simulink model "dual_RigidBodyDynamics"  (R2016a)
settings: Solver=VariableStepAuto  StartTime=0  StopTime=10  FixedStep=1  RelTol=1e-3
settings Model: Creator=viav_gi  LastModifiedBy=shriyahazra

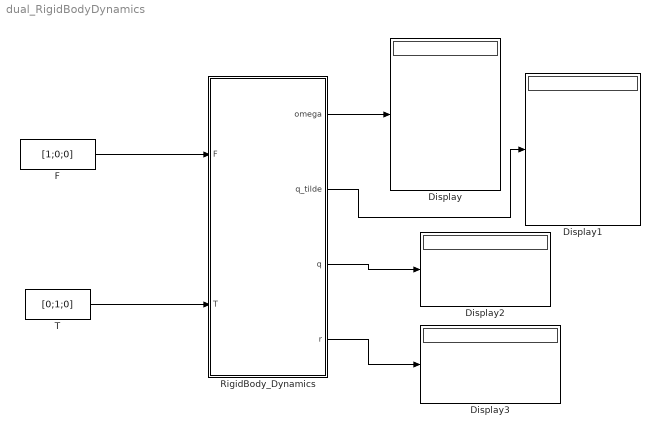
== system dual_RigidBodyDynamics ==
  Display{,1..3} (4 alike) : Display
  F : Constant  Value=[1;0;0]  VectorParams1D=off
  RigidBody_Dynamics : Subsystem  mask{r0=[0;0;0], v0=[0;0;0], m0=1, q0=[0;0;0;1], w0=[0;0;0], J0=eye(3)}
      mask prompts: r0 "Initial position (m) in inertial reference frame, [3,1]"; v0 "Initial velocity (m/s) in inertial reference frame, [3,1]"; m0 "Initial mass (kg), [1,1]"; q0 "Initial quaternion defining the orientation in body reference frame [4,1]"; w0 "Initial angular velocity (rad/s) in body reference frame, [3,1]"; J0 "Initial Inertia matrix (kg*m2),  [3,3]"
  T : Constant  Value=[0;1;0]  VectorParams1D=off
  wires:
  T/1 -> RigidBody_Dynamics/2(T)
  RigidBody_Dynamics/1(omega) -> Display/1
  RigidBody_Dynamics/2("q_tilde ") -> Display1/1
  RigidBody_Dynamics/3(q) -> Display2/1
  RigidBody_Dynamics/4(r) -> Display3/1
  F/1 -> RigidBody_Dynamics/1(F)

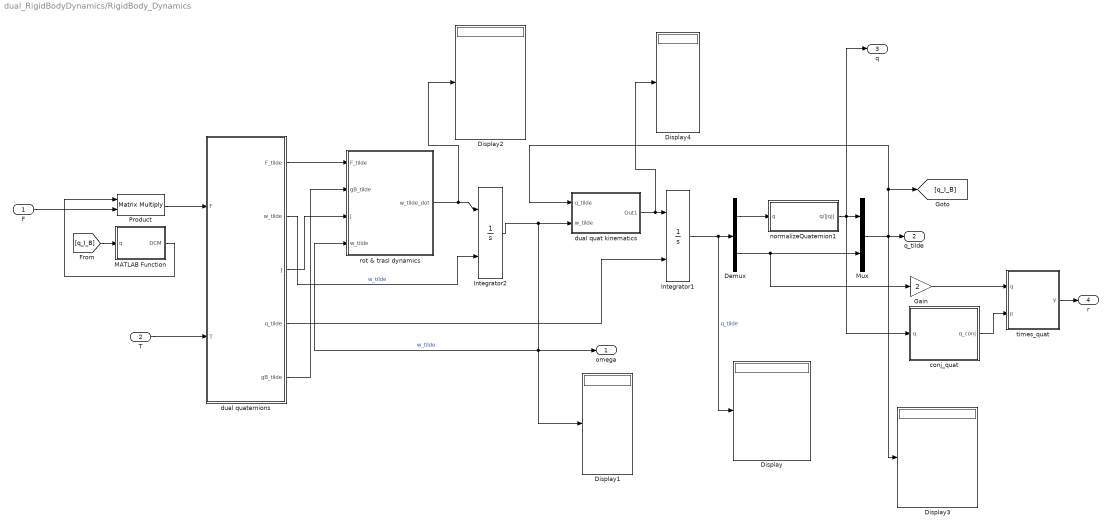
== system dual_RigidBodyDynamics/RigidBody_Dynamics ==
  F : Inport
  T : Inport  Port=2
  Demux : Demux  Outputs=2
  Display{,1..4} (5 alike) : Display
  Gain : Gain  Gain=2
  Integrator1 : Integrator  InitialConditionSource=external  InitialCondition=[0;0;0;1;0;0;0;0]
  Integrator2 : Integrator  InitialConditionSource=external  InitialCondition=[w0;0;0;0;0;0]
  MATLAB Function : MATLAB Function  TreatAsAtomicUnit=on
  Mux : Mux  Inputs=[4,4]
  Product : Product  Multiplication=Matrix(*)
  conj_quat : MATLAB Function  TreatAsAtomicUnit=on
  dual quat kinematics : Subsystem
  dual quaternions : Subsystem
  normalizeQuaternion1 : Subsystem  mask(normalizeQuaternion){}
      mask help:
      | This block is normalizing a quaternion. It changes a any quaternion into a
      | unit quaternion.
      |
      | Input:
      | 1) four dimensional quaternion
      |
      | Output:
      | 1) four dimensional unit quaternion
      mask Help: web(which('HPS_mathematics_lib-normalizeQuaternion.html'),'-helpbrowser')
  rot & trasl dynamics : Subsystem
  times_quat : MATLAB Function  TreatAsAtomicUnit=on
  omega : Outport
  "q_tilde " : Outport  Port=2
  q : Outport  Port=3
  r : Outport  Port=4
  wires:
  T/1 -> dual quaternions/2(T)
  dual quaternions/1(F_tilde) -> rot & trasl dynamics/1(F_tilde)
  dual quaternions/5(gB_tilde) -> rot & trasl dynamics/2(gB_tilde)
  dual quaternions/3(J) -> rot & trasl dynamics/3(J)
  rot & trasl dynamics/1(w_tilde_dot) -> Display2/1, Integrator2/1
  Integrator2/1 -> Display1/1, omega/1, rot & trasl dynamics/4(w_tilde), dual quat kinematics/2(w_tilde)  "w_tilde"
  dual quat kinematics/1(Out1) -> Display4/1, Integrator1/1
  dual quaternions/2(w_tilde) -> Integrator2/2  "w_tilde"
  Demux/1 -> normalizeQuaternion1/1(q)
  Integrator1/1 -> Display/1, Demux/1  "q_tilde"
  normalizeQuaternion1/1(q/||q||) -> conj_quat/1(q), Mux/1, q/1
  Demux/2 -> Gain/1, Mux/2
  Mux/1 -> [q_I_B], dual quat kinematics/1(q_tilde), Display3/1, "q_tilde "/1
  dual quaternions/4(q_tilde) -> Integrator1/2
  Gain/1 -> times_quat/1(q)
  times_quat/1(y) -> r/1
  [q_I_B] -> MATLAB Function/1(q)
  MATLAB Function/1(DCM) -> Product/1
  F/1 -> Product/2
  Product/1 -> dual quaternions/1(F)
  conj_quat/1(q_conj) -> times_quat/2(p)

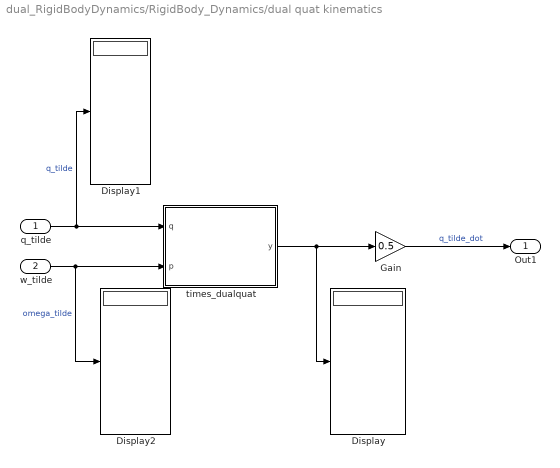
== system dual_RigidBodyDynamics/RigidBody_Dynamics/dual quat kinematics ==
  q_tilde : Inport
  w_tilde : Inport  Port=2
  Display : Display
  Display1 : Display
  Display2 : Display
  Gain : Gain  Gain=0.5
  times_dualquat : MATLAB Function  TreatAsAtomicUnit=on
  Out1 : Outport
  wires:
  q_tilde/1 -> Display1/1, times_dualquat/1(q)  "q_tilde"
  w_tilde/1 -> Display2/1, times_dualquat/2(p)  "omega_tilde"
  times_dualquat/1(y) -> Display/1, Gain/1
  Gain/1 -> Out1/1  "q_tilde_dot"

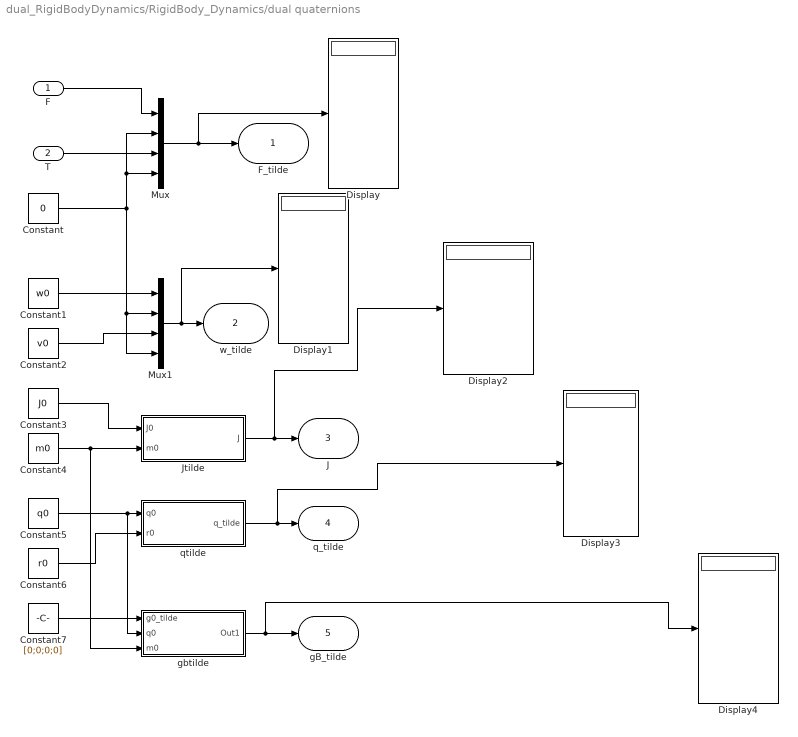
== system dual_RigidBodyDynamics/RigidBody_Dynamics/dual quaternions ==
  F : Inport
  T : Inport  Port=2
  Constant : Constant  Value=0
  Constant1 : Constant  Value=w0  VectorParams1D=off
  Constant2 : Constant  Value=v0  VectorParams1D=off
  Constant3 : Constant  Value=J0
  Constant4 : Constant  Value=m0  VectorParams1D=off
  Constant5 : Constant  Value=q0  VectorParams1D=off
  Constant6 : Constant  Value=r0  VectorParams1D=off
  Constant7 : Constant  Value=[0;0;0;0]  VectorParams1D=off
  Display{,1..4} (5 alike) : Display
  Jtilde : Subsystem
  Mux : Mux
  Mux1 : Mux
  gbtilde : Subsystem
  qtilde : Subsystem
  F_tilde : Outport
  w_tilde : Outport  Port=2
  J : Outport  Port=3
  q_tilde : Outport  Port=4
  gB_tilde : Outport  Port=5
  wires:
  F/1 -> Mux/1
  Constant/1 -> Mux1/2, Mux1/4, Mux/2, Mux/4
  Constant3/1 -> Jtilde/1(J0)
  Constant1/1 -> Mux1/1
  Constant5/1 -> gbtilde/2("q0 "), qtilde/1(q0)
  Mux/1 -> Display/1, F_tilde/1
  Mux1/1 -> Display1/1, w_tilde/1
  Constant2/1 -> Mux1/3
  Constant7/1 -> gbtilde/1(g0_tilde)
  Constant6/1 -> qtilde/2(r0)
  Constant4/1 -> Jtilde/2("m0 "), gbtilde/3(m0)
  T/1 -> Mux/3
  Jtilde/1(J) -> Display2/1, J/1
  qtilde/1(q_tilde) -> Display3/1, q_tilde/1
  gbtilde/1(Out1) -> Display4/1, gB_tilde/1

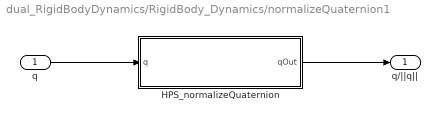
== system dual_RigidBodyDynamics/RigidBody_Dynamics/normalizeQuaternion1 ==
  q : Inport
  HPS_normalizeQuaternion : MATLAB Function  TreatAsAtomicUnit=on
  q/||q|| : Outport
  wires:
  q/1 -> HPS_normalizeQuaternion/1(q)
  HPS_normalizeQuaternion/1(qOut) -> q/||q||/1

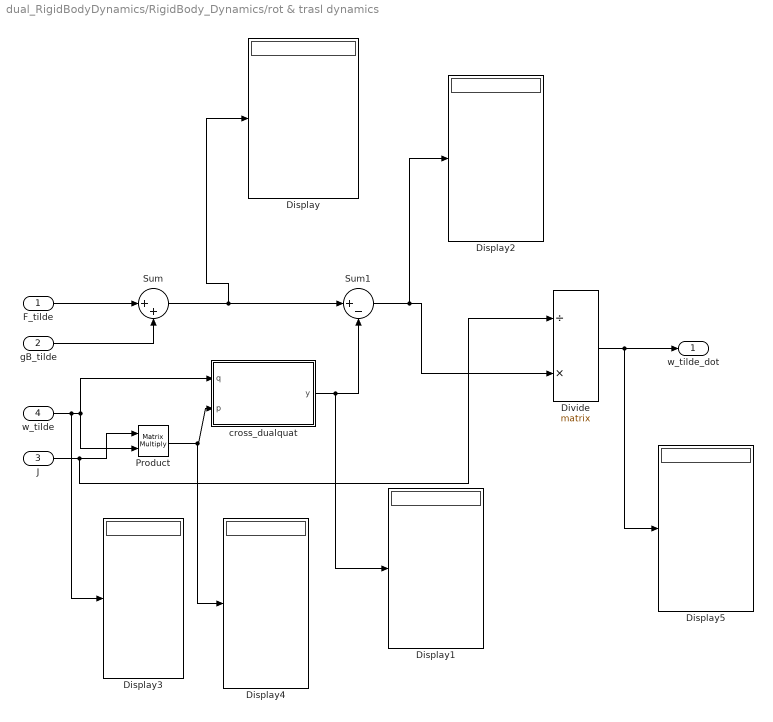
== system dual_RigidBodyDynamics/RigidBody_Dynamics/rot & trasl dynamics ==
  F_tilde : Inport
  gB_tilde : Inport  Port=2
  J : Inport  Port=3
  w_tilde : Inport  Port=4
  Display{,1..5} (6 alike) : Display
  Divide : Product  Inputs=/*  Multiplication=Matrix(*)
  Product : Product  Multiplication=Matrix(*)
  Sum : Sum  Inputs=|++
  Sum1 : Sum  Inputs=|+-
  cross_dualquat : MATLAB Function  TreatAsAtomicUnit=on
  w_tilde_dot : Outport
  wires:
  F_tilde/1 -> Sum/1
  gB_tilde/1 -> Sum/2
  J/1 -> Divide/1, Product/1
  w_tilde/1 -> Display3/1, cross_dualquat/1(q), Product/2
  Sum/1 -> Display/1, Sum1/1
  cross_dualquat/1(y) -> Display1/1, Sum1/2
  Divide/1 -> Display5/1, w_tilde_dot/1
  Product/1 -> Display4/1, cross_dualquat/2(p)
  Sum1/1 -> Display2/1, Divide/2

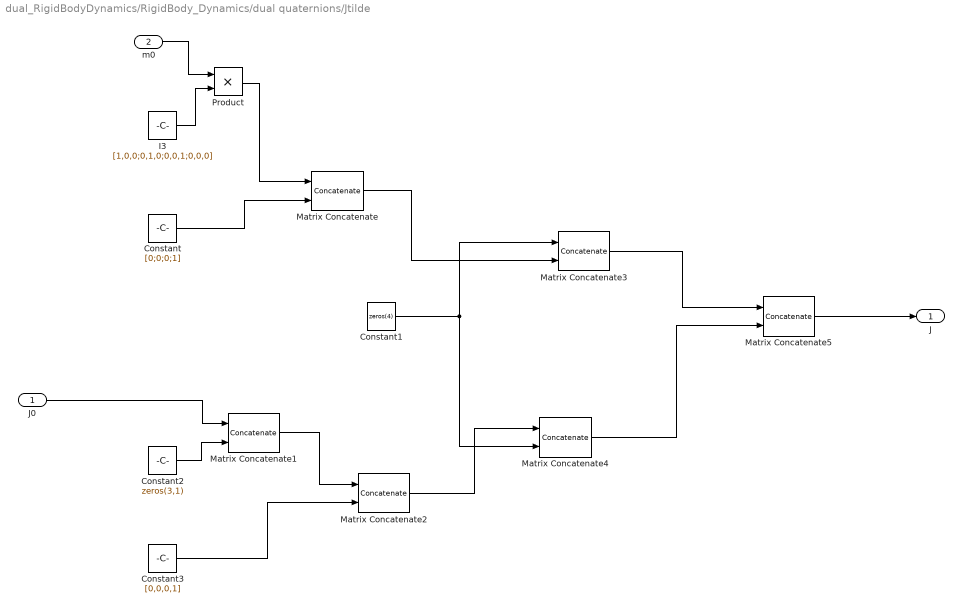
== system dual_RigidBodyDynamics/RigidBody_Dynamics/dual quaternions/Jtilde ==
  J0 : Inport
  "m0 " : Inport  Port=2
  Constant : Constant  Value=[0;0;0;1]  VectorParams1D=off
  Constant1 : Constant  Value=zeros(4)
  Constant2 : Constant  Value=zeros(3,1)
  Constant3 : Constant  Value=[0,0,0,1]  VectorParams1D=off
  I3 : Constant  Value=[1,0,0;0,1,0;0,0,1;0,0,0]
  Matrix Concatenate{,1,3..4} (4 alike) : Concatenate  Mode=Multidimensional array  ConcatenateDimension=2
  Matrix Concatenate2 : Concatenate  Mode=Multidimensional array
  Matrix Concatenate5 : Concatenate  Mode=Multidimensional array
  Product : Product
  J : Outport
  wires:
  Constant/1 -> Matrix Concatenate/2
  J0/1 -> Matrix Concatenate1/1
  Constant2/1 -> Matrix Concatenate1/2
  Matrix Concatenate1/1 -> Matrix Concatenate2/1
  Constant1/1 -> Matrix Concatenate4/2, Matrix Concatenate3/1
  Matrix Concatenate/1 -> Matrix Concatenate3/2
  Matrix Concatenate2/1 -> Matrix Concatenate4/1
  Matrix Concatenate3/1 -> Matrix Concatenate5/1
  Matrix Concatenate4/1 -> Matrix Concatenate5/2
  I3/1 -> Product/2
  Product/1 -> Matrix Concatenate/1
  Constant3/1 -> Matrix Concatenate2/2
  Matrix Concatenate5/1 -> J/1
  "m0 "/1 -> Product/1

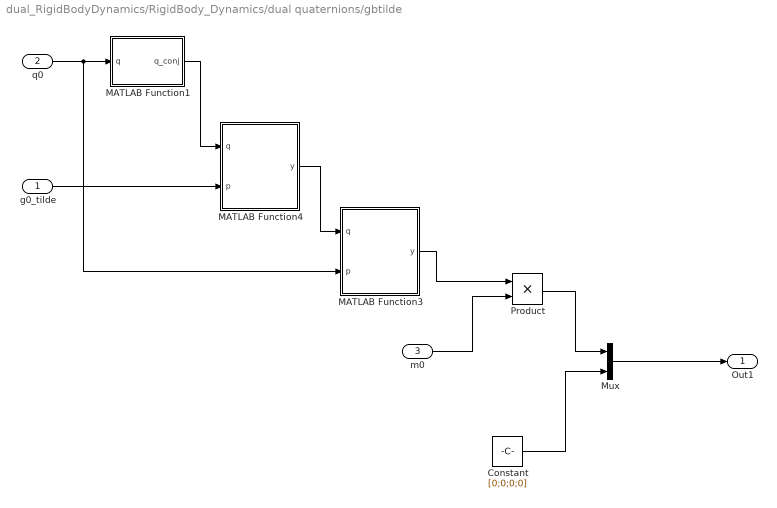
== system dual_RigidBodyDynamics/RigidBody_Dynamics/dual quaternions/gbtilde ==
  g0_tilde : Inport
  "q0 " : Inport  Port=2
  m0 : Inport  Port=3
  Constant : Constant  Value=[0;0;0;0]  VectorParams1D=off
  MATLAB Function1 : MATLAB Function  TreatAsAtomicUnit=on
  MATLAB Function3 : MATLAB Function  TreatAsAtomicUnit=on
  MATLAB Function4 : MATLAB Function  TreatAsAtomicUnit=on
  Mux : Mux  Inputs=2
  Product : Product
  Out1 : Outport
  wires:
  "q0 "/1 -> MATLAB Function3/2(p), MATLAB Function1/1(q)
  g0_tilde/1 -> MATLAB Function4/2(p)
  MATLAB Function3/1(y) -> Product/1
  Product/1 -> Mux/1
  Constant/1 -> Mux/2
  Mux/1 -> Out1/1
  MATLAB Function1/1(q_conj) -> MATLAB Function4/1(q)
  m0/1 -> Product/2
  MATLAB Function4/1(y) -> MATLAB Function3/1(q)

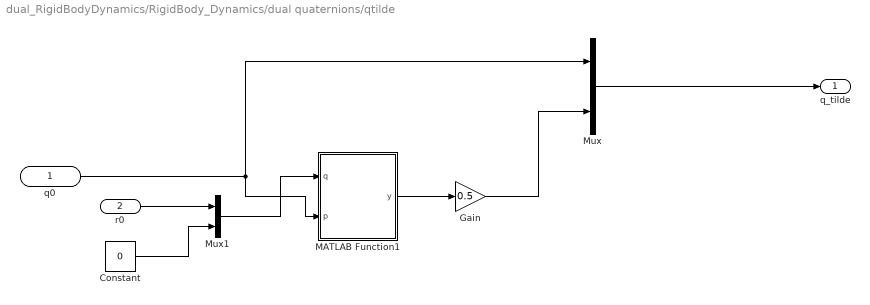
== system dual_RigidBodyDynamics/RigidBody_Dynamics/dual quaternions/qtilde ==
  q0 : Inport
  r0 : Inport  Port=2
  Constant : Constant  Value=0
  Gain : Gain  Gain=0.5
  MATLAB Function1 : MATLAB Function  TreatAsAtomicUnit=on
  Mux : Mux  Inputs=2
  Mux1 : Mux  Inputs=2
  q_tilde : Outport
  wires:
  q0/1 -> MATLAB Function1/2(p), Mux/1
  Mux/1 -> q_tilde/1
  Constant/1 -> Mux1/2
  Mux1/1 -> MATLAB Function1/1(q)
  MATLAB Function1/1(y) -> Gain/1
  r0/1 -> Mux1/1
  Gain/1 -> Mux/2

== matlab function dual_RigidBodyDynamics/RigidBody_Dynamics/dual quaternions/gbtilde/MATLAB Function1 ==
  data: q input; q_conj output
function q_conj = conj_quat(q)
%Unit quaternion conjugation

q0= q(4);
q_vect= q(1:3);

q_conj = [-q_vect; q0];

== matlab function dual_RigidBodyDynamics/RigidBody_Dynamics/dual quat kinematics/times_dualquat ==
  data: q input; y output; p input
function y = times_dualquat(q,p)
% Dual Quaternion Cross Product

q1= q(1:4);
q10= q1(4);
q1vect= q1(1:3);

p1= p(1:4);
p10= p1(4);
p1vect= p1(1:3);

q2= q(5:8);
q20= q2(4);
q2vect= q2(1:3);

p2= p(5:8);
p20= p2(4);
p2vect= p2(1:3);

y1= [q10.*p1vect + p10.*q1vect + cross(q1vect, p1vect); ...
    q10*p10 - q1vect'*p1vect];
y2= [q10.*p2vect + p20.*q1vect + cross(q1vect, p2vect); ...
    q10*p20 - q1vect'*p2vect];
y3= [q20.*p1vect + p10.*q2vect + cross(q2vect, p1vect); ...
    q20*p10 - q2vect'*p1vect];

y= [y1; y2+y3];

== matlab function dual_RigidBodyDynamics/RigidBody_Dynamics/dual quaternions/qtilde/MATLAB Function1 ==
  data: q input; y output; p input
function y = times_quat(q,p)
% Quaternion multiplication 

q0= q(4);
p0= p(4);

q_vect= q(1:3);
p_vect= p(1:3);


y = [q0.*p_vect + p0.*q_vect + cross(q_vect, p_vect); ...
    q0*p0 - sum(q_vect.*p_vect,1)];

== matlab function dual_RigidBodyDynamics/RigidBody_Dynamics/normalizeQuaternion1/HPS_normalizeQuaternion ==
  data: q input; qOut output
%----------------------------------------------------------------------------
%
%            High Performance Satellite Dynamics Simulator (HPS)
%        (c) copyright 2001 - 2008 ZARM, University of Bremen
%        (c) copyright 2008 - 2012 ZARM, University of Bremen
%        and Institute of Space Systems, DLR e.V.
%
%----------------------------------------------------------------------------
%% normalizeQuaternion()
%
% * $LastChangedBy$
% * $LastChangedRevision$
% * $LastChangedDate$
%
% *Change Record:*
%
% * 2009/10/13      - Ansgar Heidecker, initial realease
% * 2010/07/02      - Ansgar Heidecker, moved file from AF/SSB to HPS
% * 2014/10/24      - Stephen Steffes, allowed for array inputs
%
%%%
% This block normalizes a quaternion using the vector norm.
% Its basis is the embedded Matlab function
% \textit{HPS\_normalizeQuaternion.m} that is wrapped into the Simulink
% block.  If the input is a zero quaternion, the output is also a zero
% quaternion.
% 
% The inputs can be single quaternions in row or column form, or arrays
% of quaternions in column form. I.e. the size of $q$ is either $4xN$ or
% $1x4$.
% 
% *Inputs:*
% 
% * q - [4xN or 1x4] Vector or array of quaternion columns
% 
% *Returns:*
% 
% * qOut - [4xN or 1x4] Normalized quaternions with the same size as the input.
%

function qOut = HPS_normalizeQuaternion(q)
%#codegen
%#eml

    sz=size(q); %sz(1)= #rows, sz(2)= #columns
    if( (sz(1)==1 && sz(2)==4) ) % q is row vector
        n=norm(q);
        if(n~=0) % protect from div-by-0
            qOut=q/norm(q);
        else
            qOut=q;
        end
    elseif( sz(1)~=4 ) % size of q is invalid
        error('ErrorTests:convertTest','Invalid size of q.\nEither #rows of q ~= 4 or q is not a row vector with 4 cols.');
    else
        n=sqrt(sum(q.^2));
        n=n+(n==0); % protect from div-by-0
        qOut=q./(ones(4,1)*n);
    end
end

%% Reference
%
% * Wertz J.R., Spacecraft Attitude Determination and Control, Reprint
% 2002, Kluwer Academic Publishers, Appendix D

== matlab function dual_RigidBodyDynamics/RigidBody_Dynamics/dual quaternions/gbtilde/MATLAB Function3 ==
  data: q input; y output; p input
function y = times_quat(q,p)
% Quaternion multiplication 

q0= q(4);
p0= p(4);

q_vect= q(1:3);
p_vect= p(1:3);


y = [q0.*p_vect + p0.*q_vect + cross(q_vect, p_vect); ...
    q0*p0 - sum(q_vect.*p_vect,1)];

== matlab function dual_RigidBodyDynamics/RigidBody_Dynamics/dual quaternions/gbtilde/MATLAB Function4 ==
  data: q input; y output; p input
function y = times_quat(q,p)
% Quaternion multiplication 

q0= q(4);
p0= p(4);

q_vect= q(1:3);
p_vect= p(1:3);


y = [q0.*p_vect + p0.*q_vect + cross(q_vect, p_vect); ...
    q0*p0 - sum(q_vect.*p_vect,1)];

== matlab function dual_RigidBodyDynamics/RigidBody_Dynamics/rot & trasl dynamics/cross_dualquat ==
  data: q input; y output; p input
function y = cross_dualquat(q,p)
% Dual Quaternion Cross Product

q1= q(1:4);
q10= q1(4);
q1vect= q1(1:3);

p1= p(1:4);
p10= p1(4);
p1vect= p1(1:3);

q2= q(5:8);
q20= q2(4);
q2vect= q2(1:3);

p2= p(5:8);
p20= p2(4);
p2vect= p2(1:3);

y1= [q10.*p1vect + p10.*q1vect + cross(q1vect, p1vect); 0]; % q_1 x p_1
y2= [q10.*p2vect + p20.*q1vect + cross(q1vect, p2vect); 0]; % q_1 x p_2
y3= [q20.*p1vect + p10.*q2vect + cross(q2vect, p1vect); 0]; % q_2 x p_1

y= [y1; y2+y3];

== matlab function dual_RigidBodyDynamics/RigidBody_Dynamics/MATLAB Function ==
  data: q input; DCM output
% Q2DCM.m
% Function to convert quaternion to DCM.
%
% Inputs:
%     q - The quaternion to use in (vector,scalar) form
% 
% Outputs:
%     DCM - The DCM representation of q
% 
% Notes:
% See J. R. Wertz, "Spacecraft Attitude Determination and Control", 1978
% eq 12-13
function DCM = Q2DCM(q)

q=reshape(q,[],1);

qx=[0 -q(3) q(2);q(3) 0 -q(1);-q(2) q(1) 0];

DCM=(q(4)^2-dot(q(1:3),q(1:3)))*eye(3)+2*q(1:3)*q(1:3)'-2*q(4)*qx;

return

== matlab function dual_RigidBodyDynamics/RigidBody_Dynamics/conj_quat ==
  data: q input; q_conj output
function q_conj = conj_quat(q)
%Unit quaternion conjugation

q0= q(4);
q_vect= q(1:3);

q_conj = [-q_vect; q0];

== matlab function dual_RigidBodyDynamics/RigidBody_Dynamics/times_quat ==
  data: q input; y output; p input
function y = times_quat(q,p)
% Quaternion multiplication 

q0= q(4);
p0= p(4);

q_vect= q(1:3);
p_vect= p(1:3);


y = [q0.*p_vect + p0.*q_vect + cross(q_vect, p_vect); ...
    q0*p0 - sum(q_vect.*p_vect,1)];
